simulink model "hw79"  (R2021b)
settings: Solver=ode1  StartTime=0.0  StopTime=10.0  FixedStep=0.001  RelTol=1e-3
settings Model: Creator=user  LastModifiedBy=user

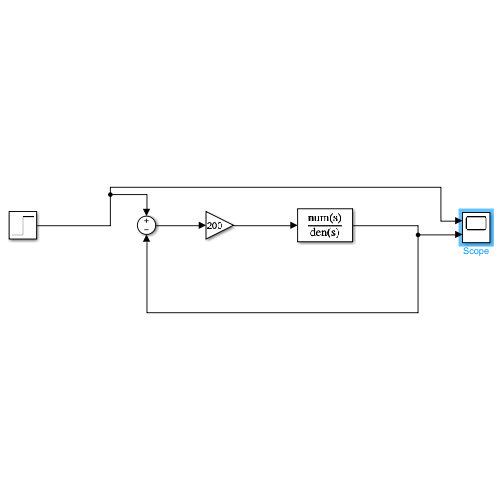
[thumbnail: Simulink's stored preview of the top-level diagram]
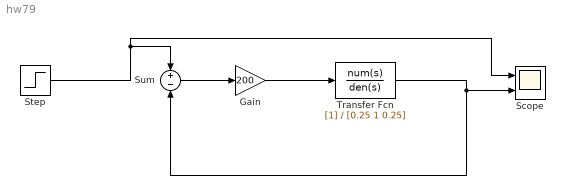
== system hw79 ==
  Gain : Gain  Gain=200
  Scope : Scope  NumInputPorts=2
  Step : Step  Time=0  SampleTime=0
  Sum : Sum  Inputs=+-
  Transfer Fcn : TransferFcn  Denominator=[0.25 1 0.25]
  wires:
  Sum/1 -> Gain/1
  Transfer Fcn/1 -> Scope/2, Sum/2
  Gain/1 -> Transfer Fcn/1
  Step/1 -> Scope/1, Sum/1
